simulink model "stateMachineModel"  (Simulink 8.6)
settings: Solver=FixedStepDiscrete  StartTime=0.0  StopTime=CONFIG.SIMULATION_TIME  FixedStep=CONFIG.Ts  RelTol=1e-3
InitFcn:
  | initSimpleSM
undefined symbols (not defined in the file): CONFIG, gain, ROBOT_DOF, sm, WBT_modelName
libraries: WBToolboxLibrary x25
settings Model: Creator=makaveli  LastModifiedBy=makaveli
settings DataIOCC: SaveFormat=Dataset  SignalLoggingSaveFormat=Dataset
settings OptimizationCC: ExpressionDepthLimit=128
settings DebuggingCC: UnderspecifiedInitializationDetection=Simplified  MergeDetectMultiDrivingBlocksExec=error  SolverPrmCheckMsg=none  FcnCallInpInsideContextMsg=EnableAllAsError  StateNameClashWarn=none
settings HardwareCC: ProdBitPerPointer=64  ProdLargestAtomicFloat=Float  ProdIntDivRoundTo=Zero  ProdEndianess=LittleEndian  ProdWordSize=64  ProdHWDeviceType=Intel->x86-64 (Windows64)
settings GRTTargetCC: GeneratePreprocessorConditionals=Use local settings  CombineOutputUpdateFcns=on  GRTInterface=off
settings ConfigComp: CovModelRefEnable=off

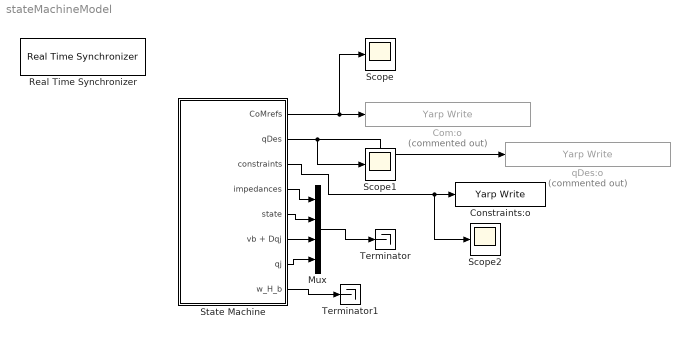
== system stateMachineModel ==
  Com:o : WBToolboxLibrary/Utilities/Yarp Write  Commented=on  portName=['/',WBT_modelName,'/comDes:o']  autoconnect=off  errorOnConnection=on
  Constraints:o : WBToolboxLibrary/Utilities/Yarp Write  portName=['/',WBT_modelName,'/constraints:o']  autoconnect=off  errorOnConnection=on
  Mux : Mux
  Real Time Synchronizer : WBToolboxLibrary/Utilities/Real Time Synchronizer  period=CONFIG.Ts
  Scope : Scope
  Scope1 : Scope
  Scope2 : Scope
  State Machine : Subsystem  Priority=-100
  Terminator : Terminator
  Terminator1 : Terminator
  qDes:o : WBToolboxLibrary/Utilities/Yarp Write  Commented=on  portName=['/',WBT_modelName,'/qDes:o']  autoconnect=off  errorOnConnection=on
  wires:
  State Machine/1(CoMrefs) -> Scope/1, Com:o/1
  State Machine/3(constraints) -> Scope2/1, Constraints:o/1
  State Machine/2(qDes) -> qDes:o/1, Scope1/1
  State Machine/7(qj) -> Mux/4
  State Machine/8(w_H_b) -> Terminator1/1
  State Machine/6(vb + Dqj) -> Mux/3
  State Machine/5(state) -> Mux/2
  State Machine/4(impedances) -> Mux/1
  Mux/1 -> Terminator/1

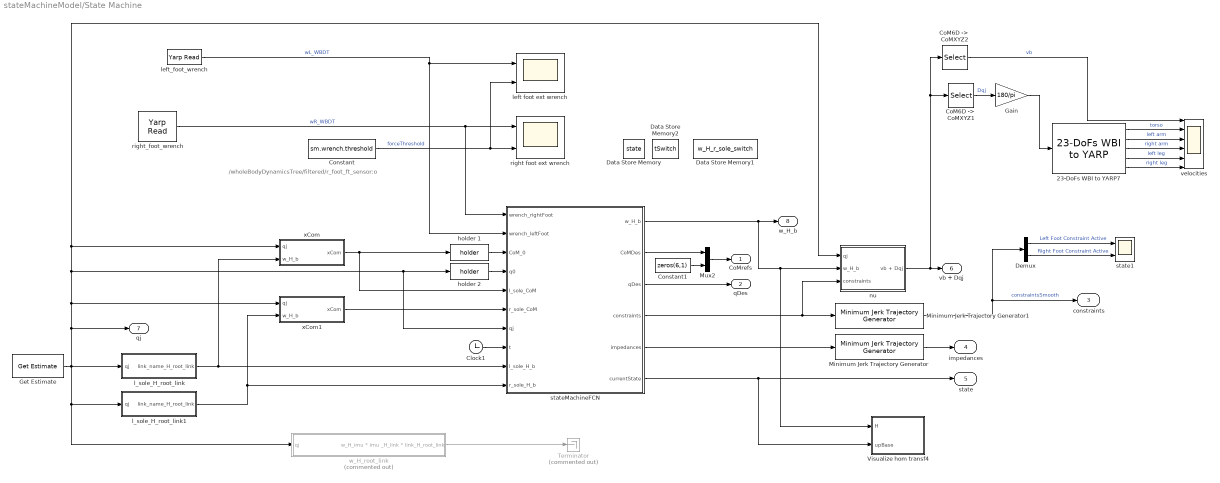
== system stateMachineModel/State Machine ==
  note: /wholeBodyDynamicsTree/filtered/r_foot_ft_sensor:o
  23-DoFs WBI to YARP7 : WBToolboxLibrary/Utilities/23-DoFs WBI to YARP
  Clock1 : Clock
  "CoM6D ->  CoMXYZ1" : Selector  InputPortWidth=ROBOT_DOF+6  IndexOptions=Index vector (dialog)  Indices=[7:ROBOT_DOF+6]  OutputSizes=1
  "CoM6D ->  CoMXYZ2" : Selector  InputPortWidth=ROBOT_DOF+6  IndexOptions=Index vector (dialog)  Indices=[1 2 3 4 5 6]  OutputSizes=1
  Constant : Constant  Value=sm.wrench.threshold
  Constant1 : Constant  Value=zeros(6,1)
  Data Store Memory : DataStoreMemory  DataStoreName=state  InitialValue=sm.stateAt0  OutDataTypeStr=double
  Data Store Memory1 : DataStoreMemory  DataStoreName=w_H_r_sole_switch  InitialValue=zeros(4)  OutDataTypeStr=double
  Data Store Memory2 : DataStoreMemory  DataStoreName=tSwitch  OutDataTypeStr=double
  Demux : Demux  Outputs=2
  Gain : Gain  Gain=180/pi
  Get Estimate : WBToolboxLibrary/wholeBodyStates/Get Estimate  estimateType=Joints Position  robotName=WBT_robotName  localName=WBT_modelName  wbiFile=WBT_wbiFilename  wbiList=WBT_wbiList
  Minimum Jerk Trajectory Generator : WBToolboxLibrary/Utilities/Minimum Jerk Trajectory Generator  externalSettlingTime=off  settlingTime=gain.SmoothingTimeImp  sampleTime=CONFIG.Ts  firstDerivatives=off  secondDerivatives=off  explicitInitialValue=off
  Minimum Jerk Trajectory Generator1 : WBToolboxLibrary/Utilities/Minimum Jerk Trajectory Generator  externalSettlingTime=off  settlingTime=smoothingTimeTransitionDynamics  sampleTime=CONFIG.Ts  firstDerivatives=off  secondDerivatives=off  explicitInitialValue=off
  Mux2 : Mux  Inputs=2
  Terminator : Terminator  Commented=on
  Visualize hom transf4 : Subsystem
  holder 1 : WBToolboxLibrary/Utilities/holder 
  holder 2 : WBToolboxLibrary/Utilities/holder 
  l_sole_H_root_link : Subsystem  mask{link_name='l_sole'}
  l_sole_H_root_link1 : Subsystem  mask{link_name='r_sole'}
  left foot ext wrench : Scope  NumInputPorts=2
  left_foot_wrench : WBToolboxLibrary/Utilities/Yarp Read  portName='/wholeBodyDynamicsTree/left_leg/cartesianEndEffectorWrench:o'  signalSize=6  blocking=off  timestamp=off  autoconnect=on  errorOnConnection=off
  nu : Subsystem
  right foot ext wrench : Scope  NumInputPorts=2
  right_foot_wrench : WBToolboxLibrary/Utilities/Yarp Read  portName='/wholeBodyDynamicsTree/right_leg/cartesianEndEffectorWrench:o'  signalSize=6  blocking=off  timestamp=off  autoconnect=on  errorOnConnection=off
  state1 : Scope  NumInputPorts=2
  stateMachineFCN : MATLAB Function  TreatAsAtomicUnit=on
  velocities : Scope  NumInputPorts=6
  w_H_root_link : Subsystem  Commented=on  mask{link_name='l_sole'}
      mask prompts: link_name "link name"
      mask help:
      | This block evaluates the homogeneous transformation between the world and the root link, i.e. ^wH_b. It assumes that the link specified by the variable 'link_name' has a constant position
      | w.r.t. an inertial frame, but it can rotate arbitrarily. This rotation is retrived from the IMU sensor.
  xCom : Subsystem
  xCom1 : Subsystem
  CoMrefs : Outport
  qDes : Outport  Port=2
  constraints : Outport  Port=3
  impedances : Outport  Port=4
  state : Outport  Port=5
  vb + Dqj : Outport  Port=6
  qj : Outport  Port=7
  w_H_b : Outport  Port=8
  wires:
  Constant/1 -> left foot ext wrench/2, right foot ext wrench/2  "forceThreshold"
  right_foot_wrench/1 -> right foot ext wrench/1, stateMachineFCN/1(wrench_rightFoot)  "wR_WBDT"
  xCom/1(xCom) -> stateMachineFCN/5(l_sole_CoM), holder 1/1
  holder 1/1 -> stateMachineFCN/3(CoM_0)
  holder 2/1 -> stateMachineFCN/4(q0)
  Clock1/1 -> stateMachineFCN/8(t)
  stateMachineFCN/3(qDes) -> qDes/1
  stateMachineFCN/2(CoMDes) -> Mux2/1
  Mux2/1 -> CoMrefs/1
  Constant1/1 -> Mux2/2
  stateMachineFCN/5(impedances) -> Minimum Jerk Trajectory Generator/1
  stateMachineFCN/6(currentState) -> state/1, Visualize hom transf4/2(upBase)
  Minimum Jerk Trajectory Generator1/1 -> Demux/1, constraints/1  "constraintsSmooth"
  stateMachineFCN/4(constraints) -> Minimum Jerk Trajectory Generator1/1, nu/3("constraints ")
  Demux/1 -> state1/1  "Left Foot Constraint Active"
  Demux/2 -> state1/2  "Right Foot Constraint Active"
  left_foot_wrench/1 -> stateMachineFCN/2(wrench_leftFoot), left foot ext wrench/1  "wL_WBDT"
  stateMachineFCN/1(w_H_b) -> nu/2(w_H_b), Visualize hom transf4/1(H), w_H_b/1
  Get Estimate/1 -> l_sole_H_root_link1/1(qj), w_H_root_link/1(qj), l_sole_H_root_link/1(qj), nu/1(qj), xCom/1(qj), stateMachineFCN/7(qj), holder 2/1, xCom1/1(qj), qj/1
  xCom1/1(xCom) -> stateMachineFCN/6(r_sole_CoM)
  nu/1(vb + Dqj) -> "CoM6D ->  CoMXYZ1"/1, "CoM6D ->  CoMXYZ2"/1, vb + Dqj/1
  Minimum Jerk Trajectory Generator/1 -> impedances/1
  "CoM6D ->  CoMXYZ2"/1 -> velocities/1  "vb"
  "CoM6D ->  CoMXYZ1"/1 -> Gain/1  "Dqj"
  23-DoFs WBI to YARP7/1 -> velocities/2  "torso"
  23-DoFs WBI to YARP7/2 -> velocities/3  "left arm"
  23-DoFs WBI to YARP7/3 -> velocities/4  "right arm"
  23-DoFs WBI to YARP7/4 -> velocities/5  "left leg"
  23-DoFs WBI to YARP7/5 -> velocities/6  "right leg"
  Gain/1 -> 23-DoFs WBI to YARP7/1
  l_sole_H_root_link/1(link_name_H_root_link) -> stateMachineFCN/9(l_sole_H_b), xCom/2(w_H_b)
  w_H_root_link/1(w_H_imu * imu _H_link * link_H_root_link) -> Terminator/1
  l_sole_H_root_link1/1(link_name_H_root_link) -> stateMachineFCN/10(r_sole_H_b), xCom1/2(w_H_b)

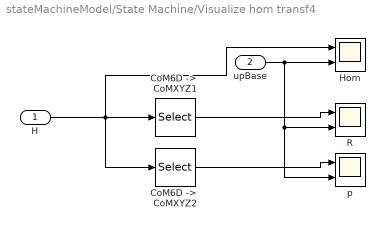
== system stateMachineModel/State Machine/Visualize hom transf4 ==
  H : Inport
  upBase : Inport  Port=2
  "CoM6D ->  CoMXYZ1" : Selector  NumberOfDimensions=2  InputPortWidth=7  IndexOptions=Index vector (dialog),Index vector (dialog)  Indices=[1 2 3],[1 2 3]  OutputSizes=1,1
  "CoM6D ->  CoMXYZ2" : Selector  NumberOfDimensions=2  InputPortWidth=7  IndexOptions=Index vector (dialog),Index vector (dialog)  Indices=[1 2 3],[4]  OutputSizes=1,1
  Hom : Scope  NumInputPorts=2
  R : Scope  NumInputPorts=2
  p : Scope  NumInputPorts=2
  wires:
  "CoM6D ->  CoMXYZ1"/1 -> R/1
  "CoM6D ->  CoMXYZ2"/1 -> p/1
  H/1 -> "CoM6D ->  CoMXYZ2"/1, Hom/1, "CoM6D ->  CoMXYZ1"/1
  upBase/1 -> p/2, R/2, Hom/2

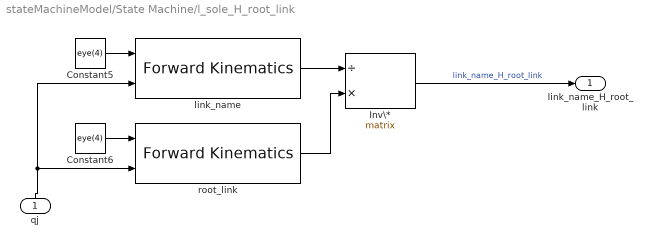
== system stateMachineModel/State Machine/l_sole_H_root_link ==
  qj : Inport
  Constant5 : Constant  Value=eye(4)
  Constant6 : Constant  Value=eye(4)
  Inv\* : Product  Inputs=/*  Multiplication=Matrix(*)
  link_name : WBToolboxLibrary/wholeBodyModel/Kinematics/Forward Kinematics  frameName=link_name  robotName=WBT_robotName  localName=WBT_modelName  wbiFile=WBT_wbiFilename  wbiList=WBT_wbiList
  root_link : WBToolboxLibrary/wholeBodyModel/Kinematics/Forward Kinematics  frameName='root_link'  robotName=WBT_robotName  localName=WBT_modelName  wbiFile=WBT_wbiFilename  wbiList=WBT_wbiList
  link_name_H_root_link : Outport
  wires:
  Constant5/1 -> link_name/1
  Inv\*/1 -> link_name_H_root_link/1  "link_name_H_root_link"
  link_name/1 -> Inv\*/1
  Constant6/1 -> root_link/1
  qj/1 -> link_name/2, root_link/2
  root_link/1 -> Inv\*/2

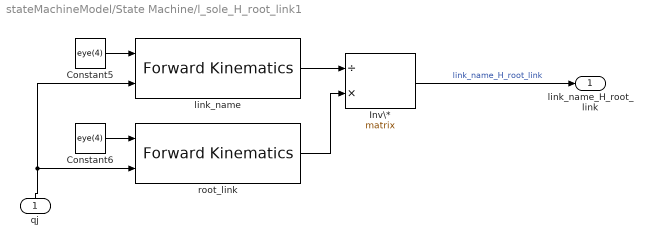
== system stateMachineModel/State Machine/l_sole_H_root_link1 ==
  qj : Inport
  Constant5 : Constant  Value=eye(4)
  Constant6 : Constant  Value=eye(4)
  Inv\* : Product  Inputs=/*  Multiplication=Matrix(*)
  link_name : WBToolboxLibrary/wholeBodyModel/Kinematics/Forward Kinematics  frameName=link_name  robotName=WBT_robotName  localName=WBT_modelName  wbiFile=WBT_wbiFilename  wbiList=WBT_wbiList
  root_link : WBToolboxLibrary/wholeBodyModel/Kinematics/Forward Kinematics  frameName='root_link'  robotName=WBT_robotName  localName=WBT_modelName  wbiFile=WBT_wbiFilename  wbiList=WBT_wbiList
  link_name_H_root_link : Outport
  wires:
  Constant5/1 -> link_name/1
  Inv\*/1 -> link_name_H_root_link/1  "link_name_H_root_link"
  link_name/1 -> Inv\*/1
  Constant6/1 -> root_link/1
  qj/1 -> link_name/2, root_link/2
  root_link/1 -> Inv\*/2

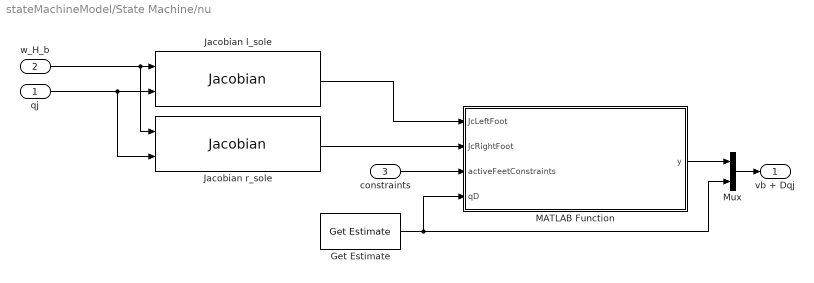
== system stateMachineModel/State Machine/nu ==
  qj : Inport
  w_H_b : Inport  Port=2
  "constraints " : Inport  Port=3
  Get Estimate : WBToolboxLibrary/wholeBodyStates/Get Estimate  estimateType=Joints Velocity  robotName=WBT_robotName  localName=WBT_modelName  wbiFile=WBT_wbiFilename  wbiList=WBT_wbiList
  Jacobian l_sole : WBToolboxLibrary/wholeBodyModel/Jacobians/Jacobian  frameName='l_sole'  robotName=WBT_robotName  localName=WBT_modelName  wbiFile=WBT_wbiFilename  wbiList=WBT_wbiList
  Jacobian r_sole : WBToolboxLibrary/wholeBodyModel/Jacobians/Jacobian  frameName='r_sole'  robotName=WBT_robotName  localName=WBT_modelName  wbiFile=WBT_wbiFilename  wbiList=WBT_wbiList
  MATLAB Function : MATLAB Function  TreatAsAtomicUnit=on
  Mux : Mux  Inputs=2
  vb + Dqj : Outport
  wires:
  Get Estimate/1 -> MATLAB Function/4(qD), Mux/2
  Mux/1 -> vb + Dqj/1
  Jacobian r_sole/1 -> MATLAB Function/2(JcRightFoot)
  "constraints "/1 -> MATLAB Function/3(activeFeetConstraints)
  MATLAB Function/1(y) -> Mux/1
  Jacobian l_sole/1 -> MATLAB Function/1(JcLeftFoot)
  qj/1 -> Jacobian r_sole/2, Jacobian l_sole/2
  w_H_b/1 -> Jacobian r_sole/1, Jacobian l_sole/1

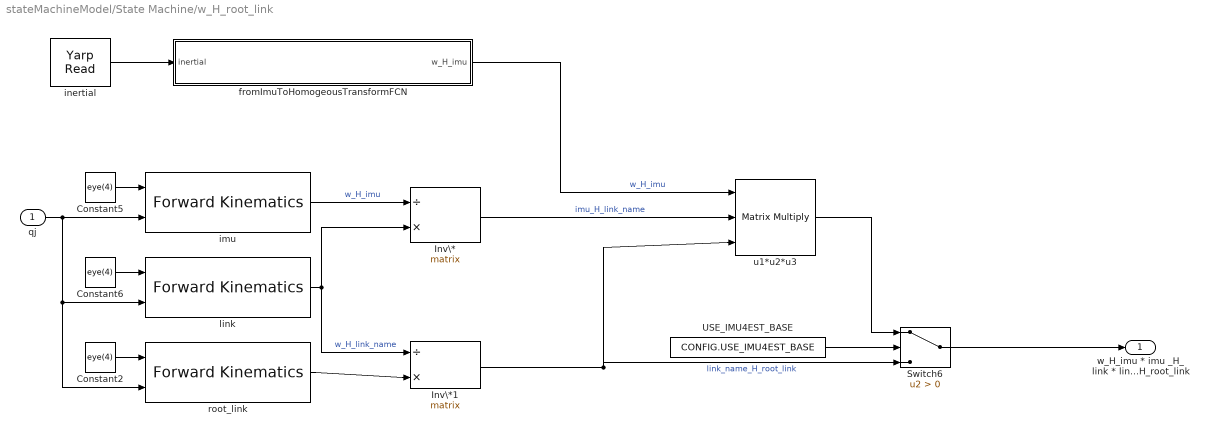
== system stateMachineModel/State Machine/w_H_root_link ==
  qj : Inport
  Constant2 : Constant  Value=eye(4)
  Constant5 : Constant  Value=eye(4)
  Constant6 : Constant  Value=eye(4)
  Inv\* : Product  Inputs=/*  Multiplication=Matrix(*)
  Inv\*1 : Product  Inputs=/*  Multiplication=Matrix(*)
  Switch6 : Switch  Criteria=u2 > Threshold
  USE_IMU4EST_BASE : Constant  Value=CONFIG.USE_IMU4EST_BASE
  fromImuToHomogeousTransformFCN : MATLAB Function  TreatAsAtomicUnit=on
  imu : WBToolboxLibrary/wholeBodyModel/Kinematics/Forward Kinematics  frameName='imu'  robotName=WBT_robotName  localName=WBT_modelName  wbiFile=WBT_wbiFilename  wbiList=WBT_wbiList
  inertial : WBToolboxLibrary/Utilities/Yarp Read  portName='/icub/inertial'  signalSize=12  blocking=off  timestamp=off  autoconnect=on  errorOnConnection=off
  link : WBToolboxLibrary/wholeBodyModel/Kinematics/Forward Kinematics  frameName=link_name  robotName=WBT_robotName  localName=WBT_modelName  wbiFile=WBT_wbiFilename  wbiList=WBT_wbiList
  root_link : WBToolboxLibrary/wholeBodyModel/Kinematics/Forward Kinematics  frameName='root_link'  robotName=WBT_robotName  localName=WBT_modelName  wbiFile=WBT_wbiFilename  wbiList=WBT_wbiList
  u1*u2*u3 : Product  Inputs=***  Multiplication=Matrix(*)
  w_H_imu * imu _H_link * link_H_root_link : Outport
  wires:
  Constant5/1 -> imu/1
  Inv\*/1 -> u1*u2*u3/2  "imu_H_link_name"
  imu/1 -> Inv\*/1  "w_H_imu"
  Constant6/1 -> link/1
  Inv\*1/1 -> u1*u2*u3/3, Switch6/3  "link_name_H_root_link"
  link/1 -> Inv\*/2, Inv\*1/1  "w_H_link_name"
  inertial/1 -> fromImuToHomogeousTransformFCN/1(inertial)
  fromImuToHomogeousTransformFCN/1(w_H_imu) -> u1*u2*u3/1  "w_H_imu"
  Switch6/1 -> w_H_imu * imu _H_link * link_H_root_link/1
  USE_IMU4EST_BASE/1 -> Switch6/2
  u1*u2*u3/1 -> Switch6/1
  Constant2/1 -> root_link/1
  qj/1 -> root_link/2, link/2, imu/2
  root_link/1 -> Inv\*1/2

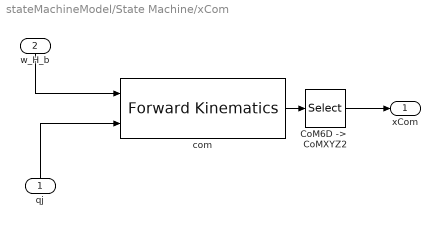
== system stateMachineModel/State Machine/xCom ==
  qj : Inport
  w_H_b : Inport  Port=2
  "CoM6D ->  CoMXYZ2" : Selector  NumberOfDimensions=2  InputPortWidth=7  IndexOptions=Index vector (dialog),Index vector (dialog)  Indices=[1 2 3],[4]  OutputSizes=1,1
  com : WBToolboxLibrary/wholeBodyModel/Kinematics/Forward Kinematics  frameName='com'  robotName=WBT_robotName  localName=WBT_modelName  wbiFile=WBT_wbiFilename  wbiList=WBT_wbiList
  xCom : Outport
  wires:
  qj/1 -> com/2
  "CoM6D ->  CoMXYZ2"/1 -> xCom/1
  com/1 -> "CoM6D ->  CoMXYZ2"/1
  w_H_b/1 -> com/1

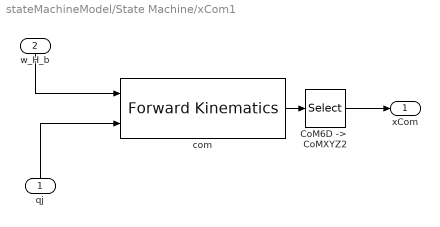
== system stateMachineModel/State Machine/xCom1 ==
  qj : Inport
  w_H_b : Inport  Port=2
  "CoM6D ->  CoMXYZ2" : Selector  NumberOfDimensions=2  InputPortWidth=7  IndexOptions=Index vector (dialog),Index vector (dialog)  Indices=[1 2 3],[4]  OutputSizes=1,1
  com : WBToolboxLibrary/wholeBodyModel/Kinematics/Forward Kinematics  frameName='com'  robotName=WBT_robotName  localName=WBT_modelName  wbiFile=WBT_wbiFilename  wbiList=WBT_wbiList
  xCom : Outport
  wires:
  qj/1 -> com/2
  "CoM6D ->  CoMXYZ2"/1 -> xCom/1
  com/1 -> "CoM6D ->  CoMXYZ2"/1
  w_H_b/1 -> com/1

== matlab function State Machine/w_H_root_link/fromImuToHomogeousTransformFCN ==
  data: inertial input double; w_H_imu output double; state data_store_memory double; tSwitch data_store_memory double; w_H_r_sole_switch data_store_memory double
function w_H_imu = fromImuToHomogeousTransformFCN(inertial)
%#codegen
 
w_H_imu = fromImuToHomogeousTransform(inertial);

== matlab function State Machine/nu/MATLAB Function ==
  data: JcLeftFoot input double; JcRightFoot input double; activeFeetConstraints input double; y output double; qD input double; reg parameter double
function y = fcn(JcLeftFoot,JcRightFoot,activeFeetConstraints,qD,reg)
%#codegen

Jc = [activeFeetConstraints(1)*JcLeftFoot;
      activeFeetConstraints(2)*JcRightFoot];

pinvJb = (Jc(:,1:6)'*Jc(:,1:6) + reg.pinvDampVb*eye(6))\Jc(:,1:6)';  
  
% pinvJb = pinv(Jc(:,1:6));

y = -pinvJb*Jc(:,7:end)*qD;

== matlab function State Machine/stateMachineFCN ==
  data: wrench_rightFoot input double; wrench_leftFoot input double; w_H_b output double; CoMDes output double; qDes output double; constraints output double; state data_store_memory double; CoM_0 input double; q0 input double; l_sole_CoM input double; r_sole_CoM input double; qj input double; t input double; l_sole_H_b input double; r_sole_H_b input double; tSwitch data_store_memory double; sm parameter double; impedances output double; gain parameter double; currentState output double; w_H_r_sole_switch data_store_memory double
function [w_H_b, CoMDes,qDes,constraints,impedances,currentState] = ...
    stateMachineFCN(wrench_rightFoot,wrench_leftFoot,CoM_0, q0, l_sole_CoM,r_sole_CoM,qj, t, l_sole_H_b, r_sole_H_b, sm,gain)
%#codegen
 
[CoMDes,qDes,constraints, currentState,impedances,w_H_b] = ...
    stateMachine(CoM_0, q0, l_sole_CoM,r_sole_CoM,qj, t, wrench_rightFoot,wrench_leftFoot,l_sole_H_b, r_sole_H_b, sm,gain);
